simulink model "verify_step_response"  (R2018a)
settings: Solver=ode4  StartTime=0.0  StopTime=10.0  FixedStep=0.01  RelTol=1e-3
libraries: simulink x1
settings Model: Creator=lenovo  LastModifiedBy=lenovo

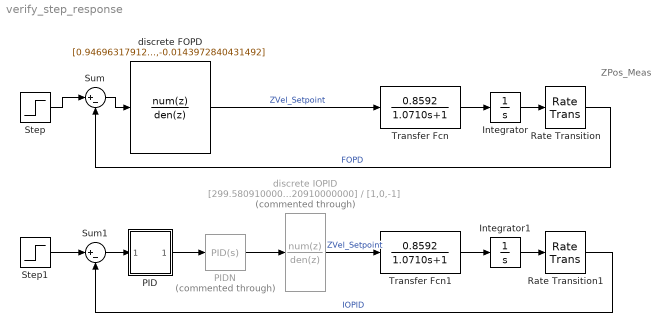
== system verify_step_response ==
  note: ZPos_Meas
  Integrator : Integrator
  Integrator1 : Integrator
  PID : Subsystem
  PIDN : simulink/Continuous/PID Controller  Commented=through  Controller=PID  TimeDomain=Continuous-time  SampleTime=-1  IntegratorMethod=Forward Euler  FilterMethod=Forward Euler  Form=Parallel  UseFilter=on  ControllerParametersSource=internal  P=1.58  I=0.182  D=1.49  N=100  InitialConditionSource=internal  InitialConditionForIntegrator=0  InitialConditionForFilter=0  ExternalReset=none  LimitOutput=off  UpperSaturationLimit=inf  LowerSaturationLimit=-inf  LinearizeAsGain=on  AntiWindupMode=none  Kb=1  TrackingMode=off  Kt=1  PParamMin=[]  PParamMax=[]  IParamMin=[]  IParamMax=[]  DParamMin=[]  DParamMax=[]  NParamMin=[]  NParamMax=[]  KbParamMin=[]  KbParamMax=[]  KtParamMin=[]  KtParamMax=[]  POutMin=[]  POutMax=[]  IOutMin=[]  IOutMax=[]  DOutMin=[]  DOutMax=[]  NOutMin=[]  NOutMax=[]  KbOutMin=[]  KbOutMax=[]  KtOutMin=[]  KtOutMax=[]  IntegratorOutMin=[]  IntegratorOutMax=[]  FilterOutMin=[]  FilterOutMax=[]  SumOutMin=[]  SumOutMax=[]  SumI1OutMin=[]  SumI1OutMax=[]  SumI2OutMin=[]  SumI2OutMax=[]  SumI3OutMin=[]  SumI3OutMax=[]  SumDOutMin=[]  SumDOutMax=[]  SaturationOutMin=[]  SaturationOutMax=[]  IntegratorContinuousStateAttributes=''  IntegratorStateMustResolveToSignalObject=off  IntegratorRTWStateStorageClass=Auto  FilterContinuousStateAttributes=''  FilterStateMustResolveToSignalObject=off  FilterRTWStateStorageClass=Auto  DifferentiatorICPrevScaledInput=0  DifferentiatorOutMin=[]  DifferentiatorOutMax=[]  FilterDiffOutCoefMin=[]  FilterDiffOutCoefMax=[]  SumDenOutMin=[]  SumDenOutMax=[]  SumNumOutMin=[]  SumNumOutMax=[]  ReciprocalOutMin=[]  ReciprocalOutMax=[]  DivideOutMin=[]  DivideOutMax=[]  TunerSelectOption=Transfer Function Based (PID Tuner App)
  Rate Transition : RateTransition  OutPortSampleTime=0.01
  Rate Transition1 : RateTransition  OutPortSampleTime=0.01
  Step : Step  SampleTime=0.01
  Step1 : Step  SampleTime=0.01
  Sum : Sum  Inputs=|+-
  Sum1 : Sum  Inputs=|+-
  Transfer Fcn : TransferFcn  Numerator=[0.8592]  Denominator=[1.0710 1]
  Transfer Fcn1 : TransferFcn  Numerator=[0.8592]  Denominator=[1.0710 1]
  discrete FOPD : DiscreteTransferFcn  Numerator=[0.946963179122833,-2.77792961698899,2.98392102212133,-1.40760552266944,0.267978964388861,-0.0129932830769816]  Denominator=[1,-2.94510699389959,3.17934233429781,-1.51000556757338,0.290497513211450,-0.0143972840431492]  SampleTime=0.01
  discrete IOPID : DiscreteTransferFcn  Commented=through  Numerator=[299.580910000000,-595.998180000000,296.420910000000]  Denominator=[1,0,-1]  SampleTime=0.01
  wires:
  Step/1 -> Sum/1
  Sum/1 -> discrete FOPD/1
  discrete FOPD/1 -> Transfer Fcn/1  "ZVel_Setpoint"
  Transfer Fcn/1 -> Integrator/1
  Integrator/1 -> Rate Transition/1
  Rate Transition/1 -> Sum/2  "FOPD"
  Step1/1 -> Sum1/1
  discrete IOPID/1 -> Transfer Fcn1/1  "ZVel_Setpoint"
  Sum1/1 -> PID/1(In1)
  Transfer Fcn1/1 -> Integrator1/1
  Rate Transition1/1 -> Sum1/2  "IOPID"
  Integrator1/1 -> Rate Transition1/1
  PIDN/1 -> discrete IOPID/1
  PID/1(Out1) -> PIDN/1

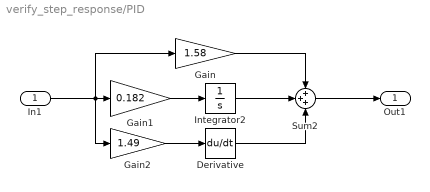
== system verify_step_response/PID ==
  In1 : Inport
  Derivative : Derivative
  Gain : Gain  Gain=1.58
  Gain1 : Gain  Gain=0.182
  Gain2 : Gain  Gain=1.49
  Integrator2 : Integrator
  Sum2 : Sum  Inputs=+++
  Out1 : Outport
  wires:
  Gain1/1 -> Integrator2/1
  In1/1 -> Gain/1, Gain2/1, Gain1/1
  Gain2/1 -> Derivative/1
  Gain/1 -> Sum2/1
  Integrator2/1 -> Sum2/2
  Derivative/1 -> Sum2/3
  Sum2/1 -> Out1/1
